simulink model "predator_prey_2024"  (R2023b)
settings: Solver=FixedStepAuto  StartTime=0.0  StopTime=100  FixedStep=0.01  RelTol=1e-3
settings Model: Creator=vaclav  LastModifiedBy=vaclav
settings OptimizationCC: ReuseModelBlockBuffer=off

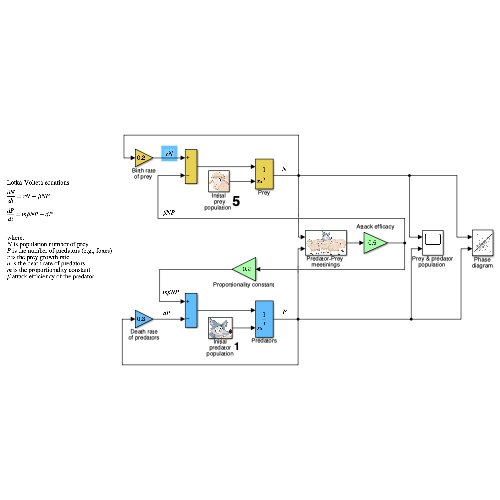
[thumbnail: Simulink's stored preview of the top-level diagram]
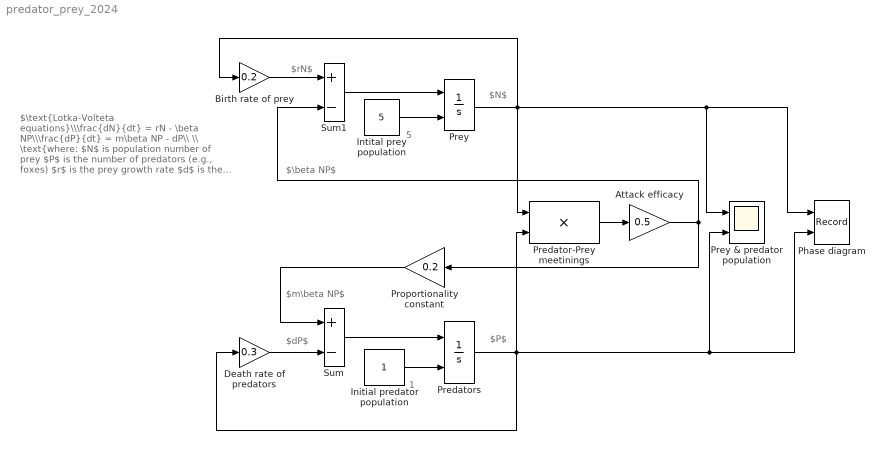
== system predator_prey_2024 ==
  note: $rN$
  note: $m\beta NP$
  note: $dP$
  note: $N$
  note: $\text{Lotka-Volteta equations}\\\frac{dN}{dt} = rN - \beta NP\\\frac{dP}{dt} = m\beta NP - dP\\ \\ \text{where: $N$ is population number of prey $P$ is the number of predators (e.g., foxes) $r$ is the prey growth rate $d$ is the death rate of predators $m$ is the proportionality constant $\beta$ attack efficiency of the predator }$
  note: 5
  note: 1
  note: $P$
  note: $\beta NP$
  Attack efficacy : Gain  Gain=0.5
  "Birth rate of prey " : Gain  Gain=0.2
  Death rate of predators : Gain  Gain=0.3
  Initial predator population : Constant
      mask Display: image('$imagefile'); % Use "Edit Image" on toolstrip to change.
  "Intital prey population " : Constant  Value=5
      mask Display: image('$imagefile'); % Use "Edit Image" on toolstrip to change.
  Phase diagram : Record  FileSettingsInternal="{\"entries\":[{\"content\":{\"excelSettings\":{\"content\":{},\"type\":\"Streamout.ExcelSettings\"}},\"type\":\"Streamout.FileSettingStorage\",\"uuid\":\"\"}],\"packageUris\":[\"http:\\/\\/schema.mathworks.com\\/mf0\\/streamout_blocks\\/R2020a\"],\"version\":\"1.0\"}"  Layout=[1 1]  SignalsInternal="{\"entries\":[{\"content\":{\"signals\":[{\"content\":{\"blockPath\":[],\"dimensions\":[1],\"domain\":\"\",\"lineColor\":\"#a2142f\",\"plots\":[ 1 ],\"port\":1,\"signalID\":1,\"signalName\":\"Prey\"},\"type\":\"RecordBlkView.Signal\",\"uuid\":\"\"},{\"content\":{\"blockPath\":[],\"dimensions\":[1],\"domain\":\"\",\"lineColor\":\"#139fff\",\"plots\":[ 1 ],\"port\":2,\"signalID\":2,\"signalName\":\"Predators\"},\"type\":\"RecordBlkView.Signal\",\"uuid\":\"\"}]},\"type\":\"RecordBlkView.InputSignals\",\"uuid\":\"\"}],\"packageUris\":[\"http:\\/\\/schema.mathworks.com\\/mf0\\/streamout_blocks\\/R2020a\"],\"version\":\"1.0\"}"  VisualizationBindings="{\"xyplotplugin\":{\"info\":[{\"series\":[{\"bindingParametersList\":[{\"parameter\":\"X-Axis\",\"signalID\":1,\"signalName\":\"Prey\"},{\"parameter\":\"Y-Axis\",\"signalID\":2,\"signalName\":\"Predators\"}],\"seriesID\":0}],\"subplotID\":1}]}}"  CompatibilityTag=XY
  Predator-Prey meetinings : Product
      mask Display: image('$imagefile'); % Use "Edit Image" on toolstrip to change.
  Predators : Integrator  InitialConditionSource=external
  Prey : Integrator  InitialConditionSource=external
  "Prey & predator population " : Scope  NumInputPorts=2
  Proportionality constant : Gain  Gain=0.2
  Sum : Sum  Inputs=+-
  Sum1 : Sum  Inputs=+-
  wires:
  Prey/1 -> "Prey & predator population "/1, Phase diagram/1, "Birth rate of prey "/1, Predator-Prey meetinings/1
  "Intital prey population "/1 -> Prey/2
  Predators/1 -> "Prey & predator population "/2, Phase diagram/2, Predator-Prey meetinings/2, Death rate of predators/1
  Initial predator population/1 -> Predators/2
  Death rate of predators/1 -> Sum/2
  Sum/1 -> Predators/1
  Proportionality constant/1 -> Sum/1
  "Birth rate of prey "/1 -> Sum1/1
  Sum1/1 -> Prey/1
  Predator-Prey meetinings/1 -> Attack efficacy/1
  Attack efficacy/1 -> Sum1/2, Proportionality constant/1
